simulink model "c63_w204_engine_sound_v6"  (R2026a)
settings: Solver=FixedStepDiscrete  StopTime=2  FixedStep=0.0001
model workspace (MAT data in the model file):
  AfterfireEgtThresholdK = 760
  CatalystReflection = -0.18
  DFCOThrottle = 0.06
  EngineIdleRPM = 700
  GearCmd = 2
  MufflerReflection = -0.42
  OverallRatio = 8.151
  RedlineRPM = 7200
  SpeedKmh = 80
  ThrottleCmd = 0.65
  V6Profile.schema = "jovi.engine_sound.v6"
  V6Profile.name = "c63_w204"
  V6Profile.display_name = "Mercedes-Benz W204 C63 AMG M156 V8"
  V6Profile.seed = 6306
  V6Profile.audio.sample_rate_hz = 96000
  V6Profile.audio.export_sample_rate_hz = 48000
  V6Profile.audio.peak_limit = 0.89
  V6Profile.engine.cylinders = 8
  V6Profile.engine.cycle_revolutions = 2
  V6Profile.engine.displacement_l = 6.208
  V6Profile.engine.bore_m = 0.1022
  V6Profile.engine.stroke_m = 0.0946
  V6Profile.engine.compression_ratio = 11.3
  V6Profile.engine.idle_rpm = 700
  V6Profile.engine.redline_rpm = 7200
  V6Profile.engine.firing_order = [1 5 4 2 6 3 7 8]
  V6Profile.engine.bank_by_cylinder = [1 2 1 2 1 2 1 2]
  V6Profile.engine.torque_rpm = [700 1500 2500 3500 4500 5000 6000 6800 7200]
  V6Profile.engine.torque_nm = [280 390 500 555 590 600 550 472 430]
  V6Profile.engine.wiebe_a = 5
  V6Profile.engine.wiebe_m = 2
  V6Profile.engine.combustion_duration_deg = 48
  V6Profile.engine.evo_deg_bbdc = 50
  V6Profile.engine.equivalent_inertia_kgm2 = 0.22
  V6Profile.driveline.gear_ratios = [4.38 2.86 1.92]
  V6Profile.driveline.final_drive = 2.85
  V6Profile.driveline.wheel_radius_m = 0.335
  V6Profile.driveline.launch_rpm = 2300
  V6Profile.driveline.max_accel_mps2 = 7.2
  V6Profile.driveline.shift_rpm = 7000
  V6Profile.driveline.shift_attack_s = 0.018
  V6Profile.driveline.shift_hold_s = 0.032
  V6Profile.driveline.shift_recovery_s = 0.075
  V6Profile.driveline.shift_settle_s = 0.055
  V6Profile.driveline.shift_min_torque = 0.22
  V6Profile.driveline.shift_reengage_gain = 1.08
  V6Profile.ecu.full_load_spark_deg = [8 16 21 24 25]
  V6Profile.ecu.spark_rpm = [700 2000 4000 6000 7200]
  V6Profile.ecu.full_load_lambda = 0.87
  V6Profile.ecu.dfco_throttle = 0.06
  V6Profile.ecu.dfco_rpm = 2200
  V6Profile.ecu.dfco_delay_s = 0.12
  V6Profile.ecu.fuel_film_tau_s = 0.18
  V6Profile.thermal.load_axis = [0.1 0.4 0.7 1]
  V6Profile.thermal.rpm_axis = [700 2000 4000 6000 7200]
  V6Profile.thermal.egt_table_k = [520  560  610  650  680; 600  660  730  790  820; 680  750  830  900  930; 720  810  900  970  1000]
  V6Profile.thermal.cooling_tau_s = 1.8
  V6Profile.thermal.gamma = 1.33
  V6Profile.thermal.gas_constant = 287
  V6Profile.blowdown.evo_pressure_pa = 350000
  V6Profile.blowdown.exhaust_temperature_k = 1050
  V6Profile.blowdown.valve_area_m2 = 0.00075
  V6Profile.blowdown.attack_s = 0.00025
  V6Profile.blowdown.fast_decay_s = 0.0018
  V6Profile.blowdown.slow_decay_s = 0.0055
  V6Profile.blowdown.fast_weight = 0.72
  V6Profile.blowdown.pulse_sharpness = 54
  V6Profile.exhaust.primary_left_m = [0.46 0.5 0.53 0.57]
  V6Profile.exhaust.primary_right_m = [0.47 0.49 0.54 0.56]
  V6Profile.exhaust.primary_diameter_m = 0.041
  V6Profile.exhaust.collector_length_m = 0.24
  V6Profile.exhaust.collector_diameter_m = 0.06
  V6Profile.exhaust.catalyst_length_m = 0.28
  V6Profile.exhaust.catalyst_diameter_m = 0.068
  V6Profile.exhaust.midpipe_length_m = 1.15
  V6Profile.exhaust.midpipe_diameter_m = 0.06
  V6Profile.exhaust.muffler_main_length_m = 0.42
  V6Profile.exhaust.muffler_bypass_length_m = 0.62
  V6Profile.exhaust.tailpipe_length_m = 0.52
  V6Profile.exhaust.tailpipe_diameter_m = 0.0635
  V6Profile.exhaust.catalyst_reflection = -0.18
  V6Profile.exhaust.catalyst_transmission = 0.72
  V6Profile.exhaust.crossover_coupling = 0.2
  V6Profile.exhaust.muffler_reflection = -0.42
  V6Profile.exhaust.tail_reflection = -0.92
  V6Profile.exhaust.loss_frequency_hz = [125 500 2000 8000 16000]
  V6Profile.exhaust.loss_db_per_m = [0.08 0.18 0.55 1.8 4.2]
  V6Profile.afterfire.egt_threshold_k = 760
  V6Profile.afterfire.minimum_rpm = 2600
  V6Profile.afterfire.overrun_duration_s = 1.25
  V6Profile.afterfire.base_interval_s = 0.029
  V6Profile.afterfire.cluster_size = 8
  V6Profile.afterfire.body_hz = [92 146 178]
  V6Profile.afterfire.metal_hz = [425 524 624 724 882]
  V6Profile.afterfire.body_gain = 0.58
  V6Profile.afterfire.metal_gain = 0.82
  V6Profile.afterfire.crack_gain = 1.78
  V6Profile.afterfire.attack_s = 0.00035
  V6Profile.afterfire.body_decay_s = 0.06
  V6Profile.afterfire.metal_decay_s = 0.018
  V6Profile.afterfire.crack_decay_s = 0.003
  V6Profile.mechanical.orders = [32 56 88]
  V6Profile.mechanical.band_gain_db = [-32 -38 -44]
  V6Profile.mechanical.noise_gain_db = -48
  V6Profile.propagation.direct_distance_m = 1
  V6Profile.propagation.ground_delay_s = 0.0048
  V6Profile.propagation.ground_gain = -0.45
  V6Profile.propagation.body_delay_s = 0.0085
  V6Profile.propagation.body_gain = -0.3
  V6SampleRateHz = 96000
  WheelRadiusM = 0.335
Description:
  | V6 C63 editable multi-rate state harness. The 96 kHz audio solver is
settings Model: DataDictionary=c63_w204_v6_params.sldd  Creator=Jovi  LastModifiedBy=Jovi
settings DataIOCC: SignalLoggingName=V6Logs

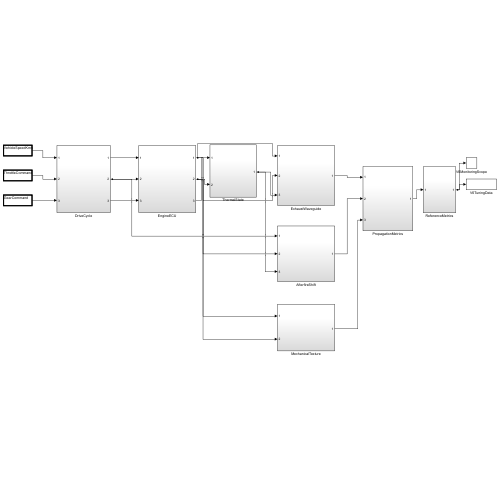
[thumbnail: Simulink's stored preview of the top-level diagram]
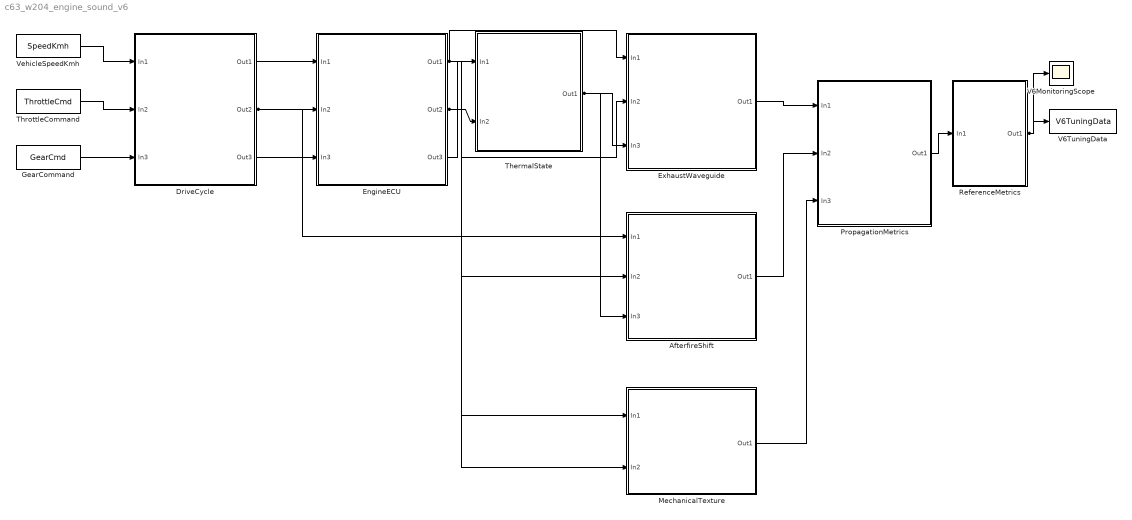
== system c63_w204_engine_sound_v6 ==
  AfterfireShift : Subsystem
  DriveCycle : Subsystem
  EngineECU : Subsystem
  ExhaustWaveguide : Subsystem
  GearCommand : Constant  Value=GearCmd
  MechanicalTexture : Subsystem
  PropagationMetrics : Subsystem
  ReferenceMetrics : Subsystem
  ThermalState : Subsystem
  ThrottleCommand : Constant  Value=ThrottleCmd
  V6MonitoringScope : Scope
  V6TuningData : ToWorkspace  VariableName=V6TuningData  SaveFormat=Structure With Time  SampleTime=-1
  VehicleSpeedKmh : Constant  Value=SpeedKmh
  wires:
  VehicleSpeedKmh/1 -> DriveCycle/1(In1)
  ThrottleCommand/1 -> DriveCycle/2(In2)
  GearCommand/1 -> DriveCycle/3(In3)
  DriveCycle/1(Out1) -> EngineECU/1(In1)
  DriveCycle/2(Out2) -> EngineECU/2(In2), AfterfireShift/1(In1)
  DriveCycle/3(Out3) -> EngineECU/3(In3)
  EngineECU/3(Out3) -> ThermalState/1(In1)
  EngineECU/2(Out2) -> ThermalState/2(In2), ExhaustWaveguide/2(In2), MechanicalTexture/2(In2)
  EngineECU/1(Out1) -> ExhaustWaveguide/1(In1), AfterfireShift/2(In2), MechanicalTexture/1(In1)
  ThermalState/1(Out1) -> ExhaustWaveguide/3(In3), AfterfireShift/3(In3)
  ExhaustWaveguide/1(Out1) -> PropagationMetrics/1(In1)
  AfterfireShift/1(Out1) -> PropagationMetrics/2(In2)
  MechanicalTexture/1(Out1) -> PropagationMetrics/3(In3)
  PropagationMetrics/1(Out1) -> ReferenceMetrics/1(In1)
  ReferenceMetrics/1(Out1) -> V6MonitoringScope/1, V6TuningData/1

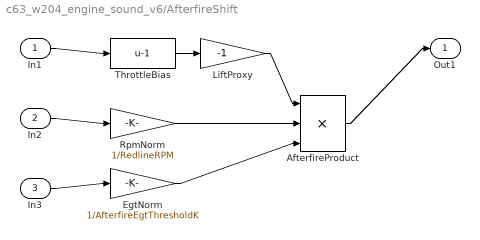
== system c63_w204_engine_sound_v6/AfterfireShift ==
  In1 : Inport
  In2 : Inport  Port=2
  In3 : Inport  Port=3
  AfterfireProduct : Product  Inputs=***
  EgtNorm : Gain  Gain=1/AfterfireEgtThresholdK
  LiftProxy : Gain  Gain=-1
  RpmNorm : Gain  Gain=1/RedlineRPM
  ThrottleBias : Bias  Bias=-1  SaturateOnIntegerOverflow=off
  Out1 : Outport
  wires:
  In1/1 -> ThrottleBias/1
  ThrottleBias/1 -> LiftProxy/1
  LiftProxy/1 -> AfterfireProduct/1
  In2/1 -> RpmNorm/1
  RpmNorm/1 -> AfterfireProduct/2
  In3/1 -> EgtNorm/1
  EgtNorm/1 -> AfterfireProduct/3
  AfterfireProduct/1 -> Out1/1

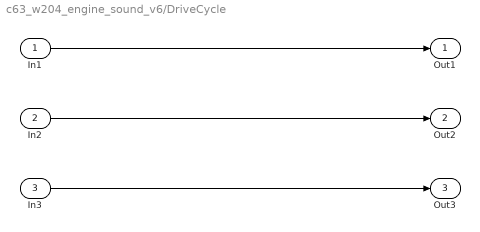
== system c63_w204_engine_sound_v6/DriveCycle ==
  In1 : Inport
  In2 : Inport  Port=2
  In3 : Inport  Port=3
  Out1 : Outport
  Out2 : Outport  Port=2
  Out3 : Outport  Port=3
  wires:
  In1/1 -> Out1/1
  In2/1 -> Out2/1
  In3/1 -> Out3/1

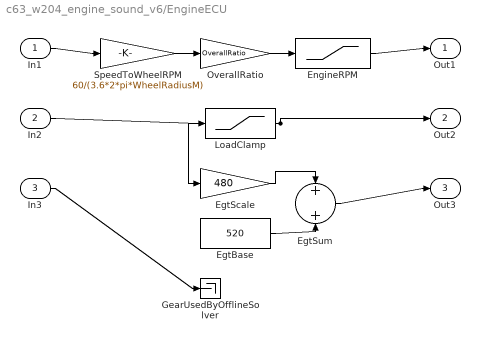
== system c63_w204_engine_sound_v6/EngineECU ==
  In1 : Inport
  In2 : Inport  Port=2
  In3 : Inport  Port=3
  EgtBase : Constant  Value=520
  EgtScale : Gain  Gain=480
  EgtSum : Sum
  EngineRPM : Saturate  UpperLimit=RedlineRPM  LowerLimit=EngineIdleRPM
  GearUsedByOfflineSolver : Terminator
  LoadClamp : Saturate  UpperLimit=1  LowerLimit=0
  OverallRatio : Gain  Gain=OverallRatio
  SpeedToWheelRPM : Gain  Gain=60/(3.6*2*pi*WheelRadiusM)
  Out1 : Outport
  Out2 : Outport  Port=2
  Out3 : Outport  Port=3
  wires:
  In1/1 -> SpeedToWheelRPM/1
  SpeedToWheelRPM/1 -> OverallRatio/1
  OverallRatio/1 -> EngineRPM/1
  EngineRPM/1 -> Out1/1
  In2/1 -> LoadClamp/1
  LoadClamp/1 -> Out2/1, EgtScale/1
  EgtScale/1 -> EgtSum/1
  EgtBase/1 -> EgtSum/2
  EgtSum/1 -> Out3/1
  In3/1 -> GearUsedByOfflineSolver/1

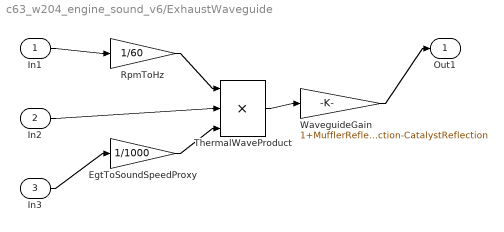
== system c63_w204_engine_sound_v6/ExhaustWaveguide ==
  In1 : Inport
  In2 : Inport  Port=2
  In3 : Inport  Port=3
  EgtToSoundSpeedProxy : Gain  Gain=1/1000
  RpmToHz : Gain  Gain=1/60
  ThermalWaveProduct : Product  Inputs=***
  WaveguideGain : Gain  Gain=1+MufflerReflection-CatalystReflection
  Out1 : Outport
  wires:
  In1/1 -> RpmToHz/1
  RpmToHz/1 -> ThermalWaveProduct/1
  In2/1 -> ThermalWaveProduct/2
  In3/1 -> EgtToSoundSpeedProxy/1
  EgtToSoundSpeedProxy/1 -> ThermalWaveProduct/3
  ThermalWaveProduct/1 -> WaveguideGain/1
  WaveguideGain/1 -> Out1/1

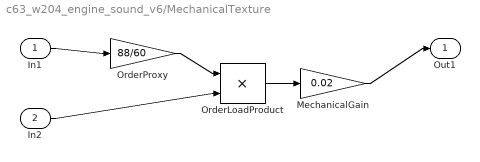
== system c63_w204_engine_sound_v6/MechanicalTexture ==
  In1 : Inport
  In2 : Inport  Port=2
  MechanicalGain : Gain  Gain=0.02
  OrderLoadProduct : Product  Inputs=**
  OrderProxy : Gain  Gain=88/60
  Out1 : Outport
  wires:
  In1/1 -> OrderProxy/1
  OrderProxy/1 -> OrderLoadProduct/1
  In2/1 -> OrderLoadProduct/2
  OrderLoadProduct/1 -> MechanicalGain/1
  MechanicalGain/1 -> Out1/1

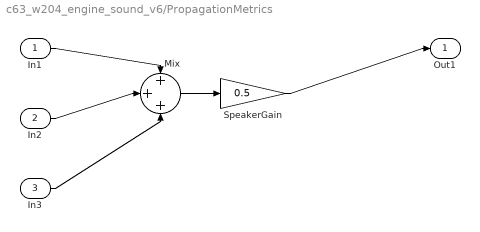
== system c63_w204_engine_sound_v6/PropagationMetrics ==
  In1 : Inport
  In2 : Inport  Port=2
  In3 : Inport  Port=3
  Mix : Sum  Inputs=+++
  SpeakerGain : Gain  Gain=0.5
  Out1 : Outport
  wires:
  In1/1 -> Mix/1
  In2/1 -> Mix/2
  In3/1 -> Mix/3
  Mix/1 -> SpeakerGain/1
  SpeakerGain/1 -> Out1/1

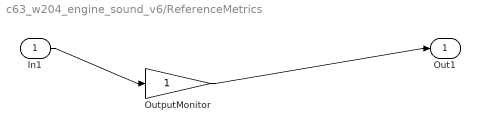
== system c63_w204_engine_sound_v6/ReferenceMetrics ==
  In1 : Inport
  OutputMonitor : Gain
  Out1 : Outport
  wires:
  In1/1 -> OutputMonitor/1
  OutputMonitor/1 -> Out1/1

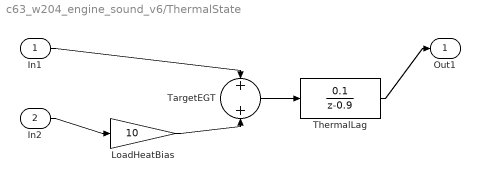
== system c63_w204_engine_sound_v6/ThermalState ==
  In1 : Inport
  In2 : Inport  Port=2
  LoadHeatBias : Gain  Gain=10
  TargetEGT : Sum
  ThermalLag : DiscreteTransferFcn  Numerator=0.1  Denominator=[1 -0.9]  SampleTime=0.001
  Out1 : Outport
  wires:
  In1/1 -> TargetEGT/1
  In2/1 -> LoadHeatBias/1
  LoadHeatBias/1 -> TargetEGT/2
  TargetEGT/1 -> ThermalLag/1
  ThermalLag/1 -> Out1/1
